simulink model "hw3_3"  (R2023a)
settings: Solver=VariableStepAuto  StartTime=0.0  StopTime=10.0  RelTol=1e-3
libraries: simulink x1
settings Model: Creator=마이컴  LastModifiedBy=마이컴

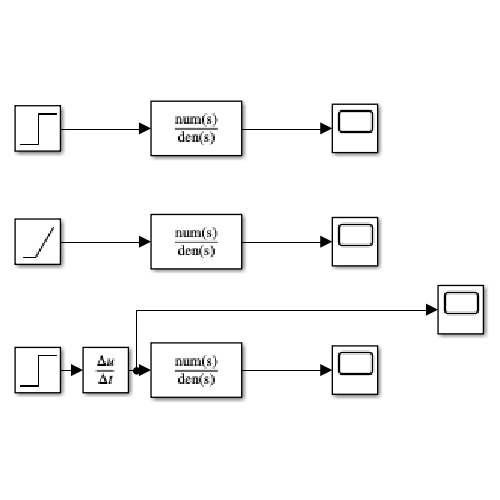
[thumbnail: Simulink's stored preview of the top-level diagram]
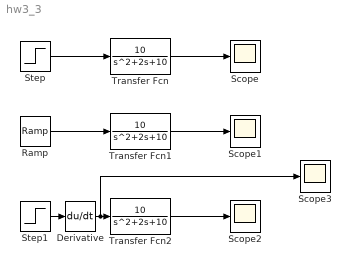
== system hw3_3 ==
  Derivative : Derivative
  Ramp : simulink/Sources/Ramp  slope=1  start=0  InitialOutput=0
  Scope{,1..3} (4 alike) : Scope
  Step : Step  Time=0  SampleTime=0
  Step1 : Step  SampleTime=0
  Transfer Fcn : TransferFcn  Numerator=[10]  Denominator=[1 2 10]
  Transfer Fcn1 : TransferFcn  Numerator=[10]  Denominator=[1 2 10]
  Transfer Fcn2 : TransferFcn  Numerator=[10]  Denominator=[1 2 10]
  wires:
  Step/1 -> Transfer Fcn/1
  Transfer Fcn/1 -> Scope/1
  Ramp/1 -> Transfer Fcn1/1
  Transfer Fcn1/1 -> Scope1/1
  Step1/1 -> Derivative/1
  Derivative/1 -> Scope3/1, Transfer Fcn2/1
  Transfer Fcn2/1 -> Scope2/1
